simulink model "askisi1"  (R2022a)
settings: Solver=ode23tb  StartTime=0.0  StopTime=1  RelTol=1e-3
libraries: spsAsynchronousMachineSIUnitsLib x1, spsNeutralLib x1, spsThreePhaseProgrammableVoltageSourceLib x1, spsVoltageMeasurementLib x1, spspowerguiLib x1
settings Model: Creator=up1053646  LastModifiedBy=CHRIS
settings DebuggingCC: UnconnectedInputMsg=warning  UnconnectedOutputMsg=warning  UnconnectedLineMsg=warning
settings RTWCC: DLArmComputeVersion=19.05

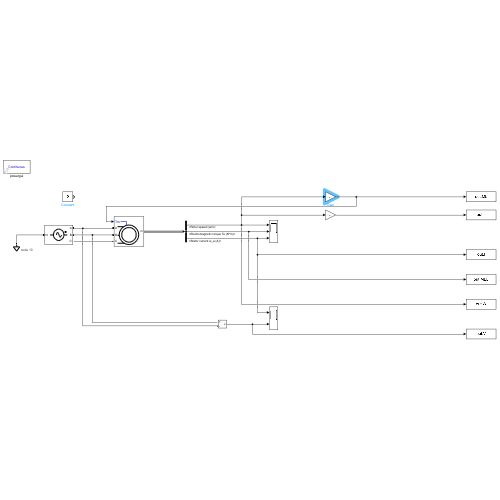
[thumbnail: Simulink's stored preview of the top-level diagram]
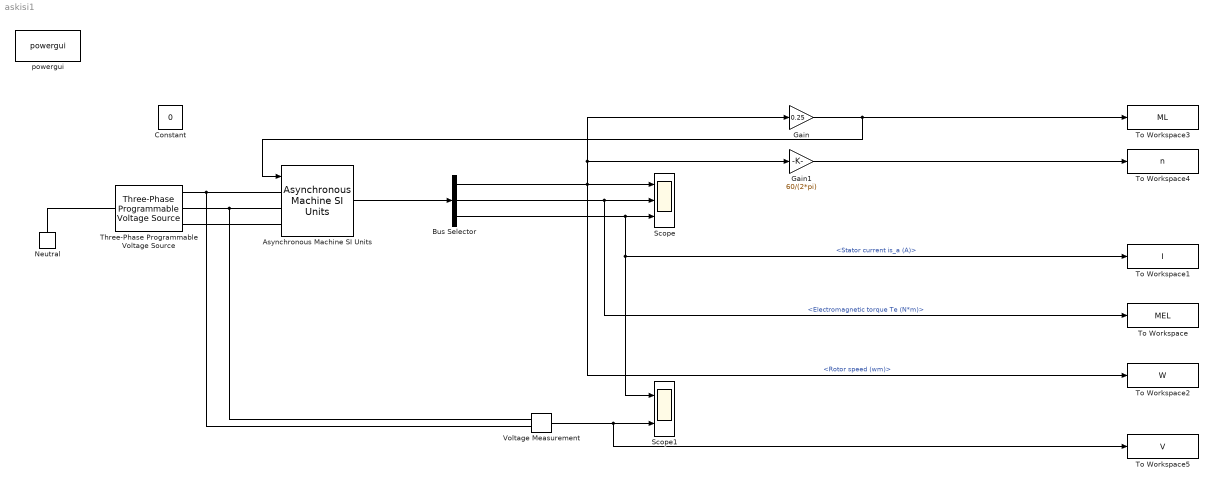
== system askisi1 ==
  Asynchronous Machine SI Units : spsAsynchronousMachineSIUnitsLib/Asynchronous Machine SI Units  RotorType=Squirrel-cage  PresetModel=No  MechanicalLoad=Torque Tm  ShowDetailedParameters=on  ReferenceFrame=Stationary  Units=SI  MeasurementBus=off  NominalParameters=[4000 400 50]  VoltageRatio=1  Stator=[1.405 0.005839]  Rotor=[1.395 0.005839]  Cage1=[0.4155 0.002066]  Cage2=[0.4168 0.0003495]  Lm=0.1722  Mechanical=[0.05 0.002985 2]  PolePairs=2  InitialConditions=[1 0 0 0 0 0 0 0]  SimulateSaturation=off  Saturation=[14.03593122, 27.81365428, 53.79336849, 72.68890987, 97.98006896, 148.6815601, 215.7428561, 302.9841135, 428.7778367 ; 230, 322, 414, 460, 506, 552, 598, 644, 690]  LoadFlowParameters=1492000  TsPowergui=0  TsBlock=-1  IterativeModel=Trapezoidal non iterative  IterativeDiscreteModel=Trapezoidal non iterative  Pmec=1.492e+006
  Bus Selector : BusSelector  OutputSignals=Mechanical.Rotor speed (wm),Mechanical.Electromagnetic torque Te (N*m),Stator measurements.Stator current is_a (A)
  Constant : Constant  Value=0
  Gain : Gain  Gain=0.25
  Gain1 : Gain  Gain=60/(2*pi)
  Neutral : spsNeutralLib/Neutral  LConnTagsString=a  NodeNumber=10
      settings: AttributesFormatString=node %<NodeNumber>  SourceProductBaseCode=PS
  Scope : Scope  NumInputPorts=3
  Scope1 : Scope  NumInputPorts=2
  Three-Phase Programmable Voltage Source : spsThreePhaseProgrammableVoltageSourceLib/Three-Phase Programmable Voltage Source  PositiveSequence="[380  0 50]"  VariationEntity=None  VariationType=Table of time-amplitude pairs  VariationTypeAlt=Step  VariationStep=0.5  VariationRate=10  VariationMagnitude=0.3  VariationFrequency=2  VariationTiming=[1 2]  VariationPhaseA=off  Amplitudes=[1 0.8 1.2 1.0]  TimeValues=[0 0.1 0.15 0.2]  HarmonicGeneration=off  HarmonicA=[3 0.2 -25 0]  HarmonicB=[2 0.15 35 2]  Timing="[0.05  3]"  BusType=swing  Pref=0  Qref=0  Qmin=-inf  Qmax=inf
  To Workspace : ToWorkspace  VariableName=MEL  SaveFormat=Timeseries  SampleTime=1e-4
  To Workspace1 : ToWorkspace  VariableName=I  SaveFormat=Timeseries  SampleTime=1e-4
  To Workspace2 : ToWorkspace  VariableName=W  SaveFormat=Timeseries  SampleTime=1e-4
  To Workspace3 : ToWorkspace  VariableName=ML  SaveFormat=Timeseries  SampleTime=1e-4
  To Workspace4 : ToWorkspace  VariableName=n  SaveFormat=Timeseries  SampleTime=1e-4
  To Workspace5 : ToWorkspace  VariableName=V  SaveFormat=Timeseries  SampleTime=1e-4
  Voltage Measurement : spsVoltageMeasurementLib/Voltage Measurement  PhasorSimulation=off  OutputType=Complex  PSBequivalent=0
  powergui : spspowerguiLib/powergui  Priority=1  SimulationMode=Continuous  SampleTime=50e-6  frequency=60  Iterations=50  frequencyindice=50  Pbase=100e6  ErrMax=1e-4  UnitsV=kV  UnitsW=MW  buscounter=0  FunctionMessages=off  echomessages=off  EnableUseOfTLC=off  CurrentSourceSwitches=off  DisableSnubberDevices=off  DisableRonSwitches=off  DisableVfSwitches=off  DisplayEquations=off  AutomaticDiscreteSolvers=off  SolverType=Tustin/Backward Euler (TBE)  Interpol=off  ExternalGateDelay=off  methode=off  Ts=100  x0status=blocks  SPID=on  SwTol=0  HookPort=off  NonlinearTolerance=1e-4  nMaxIteration=100  ContinueOnMaxIteration=off  RestoreLinks=warning  ResistiveCurrentMeasurement=off  Frange=[0:2:500]  Ylog=off  Xlog=on  ShowGrid=off  save=off  variable=ZData  structure=0  ZoomFFT=off  StartTime=0.0  cycles=1  DisplayStyle=1  fundamental=60  FreqAxis=off  MaxFrequency=1000  frequencyindicesteady=1  RmsSteady=1  display=off
  wires:
  Asynchronous Machine SI Units/1 -> Bus Selector/1
  Bus Selector/1 -> Gain/1, Gain1/1, Scope/1, To Workspace2/1  "<Rotor speed (wm)>"
  Bus Selector/2 -> To Workspace/1, Scope/2  "<Electromagnetic torque Te (N*m)>"
  Bus Selector/3 -> Scope1/1, To Workspace1/1, Scope/3  "<Stator current is_a (A)>"
  Gain/1 -> Asynchronous Machine SI Units/1, To Workspace3/1
  Gain1/1 -> To Workspace4/1
  Voltage Measurement/1 -> To Workspace5/1, Scope1/2
  connections:
  Three-Phase Programmable Voltage Source/RConn1 -- Voltage Measurement/LConn2 -- Asynchronous Machine SI Units/LConn1
  Three-Phase Programmable Voltage Source/RConn2 -- Voltage Measurement/LConn1 -- Asynchronous Machine SI Units/LConn2
  Three-Phase Programmable Voltage Source/RConn3 -- Asynchronous Machine SI Units/LConn3
  Neutral/LConn1 -- Three-Phase Programmable Voltage Source/LConn1
